simulink model "two_mass_translational"  (R2013b)
settings: Solver=ode45  StartTime=0.0  StopTime=20  RelTol=1e-3
libraries: fl_lib x9, nesl_utility x3
settings Model: Creator=User  LastModifiedBy=User

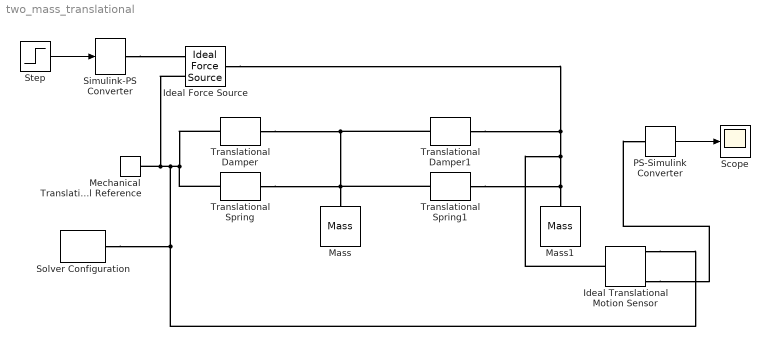
== system two_mass_translational ==
  Ideal Force Source : fl_lib/Mechanical/Mechanical Sources/Ideal Force Source  v_Log=off  f_Log=off  LocalVarNames=|v|f  LocalVarDescs=|v|f  LocalVarLogging=[0 0]
  Ideal Translational Motion Sensor : fl_lib/Mechanical/Mechanical Sensors/Ideal Translational Motion Sensor  offset=0 m  v_Log=off  f_Log=off  x_Log=off  LocalVarNames=|v|f|x  LocalVarDescs=|v|f|x  LocalVarLogging=[0 0 0]
  Mass : fl_lib/Mechanical/Translational Elements/Mass  mass=5 kg  initial_velocity=0 m/s  f_Log=off  LocalVarNames=|f  LocalVarDescs=|f  LocalVarLogging=0
  Mass1 : fl_lib/Mechanical/Translational Elements/Mass  mass=5 kg  initial_velocity=0 m/s  f_Log=off  LocalVarNames=|f  LocalVarDescs=|f  LocalVarLogging=0
  Mechanical Translational Reference : fl_lib/Mechanical/Translational Elements/Mechanical Translational Reference  f_Log=off  LocalVarNames=|f  LocalVarDescs=|f  LocalVarLogging=0
  PS-Simulink Converter : nesl_utility/PS-Simulink Converter  PhysicalDomain=network_engine_domain  SubClassName=ps_output  LeftPortType=input  RightPortType=output  PseudoPeriodic=off  Frequencies=[]  Unit=1  AffineConversion=off
  Scope : Scope
  Simulink-PS Converter : nesl_utility/Simulink-PS Converter  PhysicalDomain=network_engine_domain  SubClassName=ps_input  LeftPortType=input  RightPortType=output  PseudoPeriodic=off  Frequencies=[]  NoiseDistribution=none  NoiseParameters=[]  Unit=1  AffineConversion=off  InputFiltering=off  SimscapeFilterOrder=1  InputFilterTimeConstant=0.001  UdotUserProvided=1
  Solver Configuration : nesl_utility/Solver Configuration  PhysicalDomain=network_engine_domain  SubClassName=solver  LeftPortType=input  RightPortType=generic  Accelerate=off  Tones=[]  Harmonics=[]  SimulateNoise=off  Profile=off  UseLocalSampling=off  EnableSwitchedLinearOptims=on  FrequencyDomain=off  UseCCode=off  RelTol=0.001  AbsTol=1e-06  MinStep=1e-09  ToWorkspace=off  DoDC=off  ResidualTolerance=1e-09  UseLocalSolver=off  LocalSolverChoice=NE_BACKWARD_EULER_ADVANCER  LocalSolverSampleTime=0.001  DoFixedCost=off  MaxNonlinIter=3  MaxModeIter=2  LinearAlgebra=Sparse  DelaysMemoryBudget=1024
  Step : Step  Time=0  SampleTime=0
  Translational Damper : fl_lib/Mechanical/Translational Elements/Translational Damper  D=5 N/(m/s)  f_Log=off  v_Log=off  LocalVarNames=|f|v  LocalVarDescs=|f|v  LocalVarLogging=[0 0]
  Translational Damper1 : fl_lib/Mechanical/Translational Elements/Translational Damper  D=5 N/(m/s)  f_Log=off  v_Log=off  LocalVarNames=|f|v  LocalVarDescs=|f|v  LocalVarLogging=[0 0]
  Translational Spring : fl_lib/Mechanical/Translational Elements/Translational Spring  spr_rate=50 N/m  init_def=0 m  f_Log=off  v_Log=off  x_Log=off  LocalVarNames=|f|v|x  LocalVarDescs=|f|v|x  LocalVarLogging=[0 0 0]
  Translational Spring1 : fl_lib/Mechanical/Translational Elements/Translational Spring  spr_rate=50 N/m  init_def=0 m  f_Log=off  v_Log=off  x_Log=off  LocalVarNames=|f|v|x  LocalVarDescs=|f|v|x  LocalVarLogging=[0 0 0]
  wires:
  Step/1 -> Simulink-PS Converter/1
  PS-Simulink Converter/1 -> Scope/1
  connections:
  Translational Damper/LConn1 -- Translational Spring/LConn1 -- Ideal Translational Motion Sensor/RConn1 -- Solver Configuration/RConn1 -- Ideal Force Source/RConn2 -- Mechanical Translational Reference/LConn1
  Translational Damper/RConn1 -- Translational Damper1/LConn1 -- Translational Spring1/LConn1 -- Translational Spring/RConn1 -- Mass/LConn1
  Translational Damper1/RConn1 -- Ideal Force Source/LConn1 -- Ideal Translational Motion Sensor/LConn1 -- Translational Spring1/RConn1 -- Mass1/LConn1
  Simulink-PS Converter/RConn1 -- Ideal Force Source/RConn1
  Ideal Translational Motion Sensor/RConn3 -- PS-Simulink Converter/LConn1
